simulink model "img_edge_detect_iOS"  (R2021b)
settings: Solver=VariableStepAuto  StartTime=0.0  StopTime=10.0  RelTol=1e-3
undefined symbols (not defined in the file): none, videoinput
libraries: visionanalysis x3, imaqlib x1, visionsinks x1
settings Model: Creator=rashmibadri  LastModifiedBy=rashmibadri

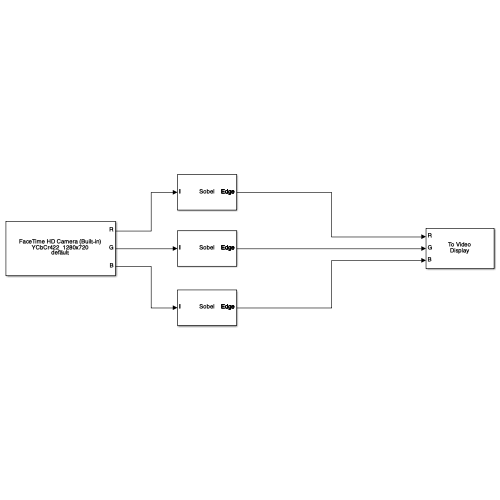
[thumbnail: Simulink's stored preview of the top-level diagram]
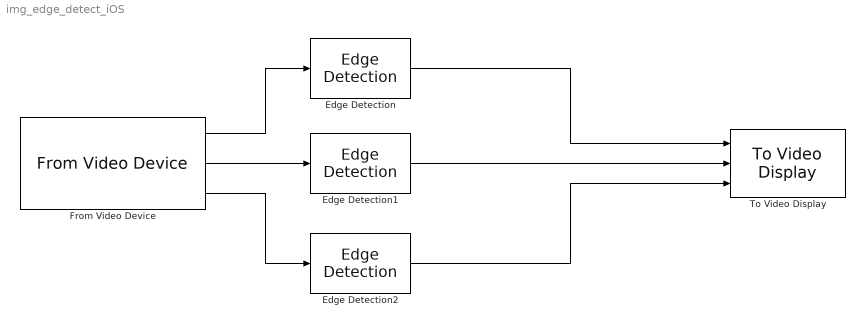
== system img_edge_detect_iOS ==
  Edge Detection : visionanalysis/Edge Detection  method=Sobel  outputType=Binary image  userDefinedThreshold=off  thresholdSource=Input port  threshold=20  thresholdTuning=4  edgeThinning=off  threshold_canny=[0.25 0.60]  autoPercent=70  sigma=1  roundingMode=Floor  overflowMode=off  prodOutputMode=Binary point scaling  prodOutputWordLength=32  prodOutputFracLength=8
      settings: SourceProductBaseCode=VP
  Edge Detection1 : visionanalysis/Edge Detection  method=Sobel  outputType=Binary image  userDefinedThreshold=off  thresholdSource=Input port  threshold=20  thresholdTuning=4  edgeThinning=off  threshold_canny=[0.25 0.60]  autoPercent=70  sigma=1  roundingMode=Floor  overflowMode=off  prodOutputMode=Binary point scaling  prodOutputWordLength=32  prodOutputFracLength=8
      settings: SourceProductBaseCode=VP
  Edge Detection2 : visionanalysis/Edge Detection  method=Sobel  outputType=Binary image  userDefinedThreshold=off  thresholdSource=Input port  threshold=20  thresholdTuning=4  edgeThinning=off  threshold_canny=[0.25 0.60]  autoPercent=70  sigma=1  roundingMode=Floor  overflowMode=off  prodOutputMode=Binary point scaling  prodOutputWordLength=32  prodOutputFracLength=8
      settings: SourceProductBaseCode=VP
  From Video Device : imaqlib/From Video Device  DeviceMenu=macvideo 1 (FaceTime HD Camera (Built-in))  Device=macvideo 1 (FaceTime HD Camera (Built-in))  ObjConstructor=videoinput('macvideo', 1)  VideoFormatMenu=YCbCr422_1280x720  VideoFormat=YCbCr422_1280x720  VideoSource=default  ROIPosition=[0 0 720 1280]  EnableHWTrigger=off  TriggerConfiguration=none/none  SampleTime=1/30  OutputPortsMode=Separate color signals  DataType=single  CanDoHWTrigger=no  ReturnedColorSpace=rgb  BlockHandle=4.0002  ROIWidth=1280  ROIHeight=720  ROIColumn=0  ROIRow=0  EngXMLPath=/Applications/MATLAB_R2021b.app/toolbox/imaq/imaq/private  DevXMLPath=/Users/rashmibadri/Documents/MATLAB/SupportPackages/R2021b/toolbox/imaq/supportpackages/genericvideo/adaptor/maci64  EngLibPath=/Applications/MATLAB_R2021b.app/toolbox/imaq/imaqblks/imaqmex/maci64  ColorSpace=rgb  BayerSensorAlignment=grbg  ImaqMode=off
  To Video Display : visionsinks/To Video Display  windowSizeMode=Normal  openAtMdlStart=on  fullScreen=off  videoWindowX=536805376  videoWindowY=536805376  saveWindowSize=off  videoWindowWidth=2147483647  videoWindowHeight=2147483647  inputColorFormat=RGB  inputType=Obsolete  imagePorts=Separate color signals  OutputDevice=On-screen video monitor  dataOrg=Column-major  isWindowOpen=off
  wires:
  Edge Detection/1 -> To Video Display/1
  From Video Device/1 -> Edge Detection/1
  From Video Device/2 -> Edge Detection1/1
  From Video Device/3 -> Edge Detection2/1
  Edge Detection1/1 -> To Video Display/2
  Edge Detection2/1 -> To Video Display/3
